simulink model "ESQUEMA"  (R2022b)
settings: Solver=VariableStepAuto  StartTime=0.0  StopTime=inf  RelTol=1e-3
libraries: dsparch4 x12, dspvision x2, dspmathops x1
settings Model: Creator=Core I5  LastModifiedBy=mluser
settings SolverCC: AlgebraicLoopSolver=TrustRegion
settings DataIOCC: ReturnWorkspaceOutputs=off
settings DebuggingCC: UnconnectedInputMsg=warning  UnconnectedOutputMsg=warning  UnconnectedLineMsg=warning  SFMachineParentedDataDiag=warning  ArithmeticOperatorsInVariantConditions=warning
settings ModelReferenceCC: EnableRefExpFcnMdlSchedulingChecks=on
settings SFSimCC: SimUseLocalCustomCode=off  CustomCodeUndefinedFunction=UseInterfaceOnly
settings RTWCC: RTWUseLocalCustomCode=off

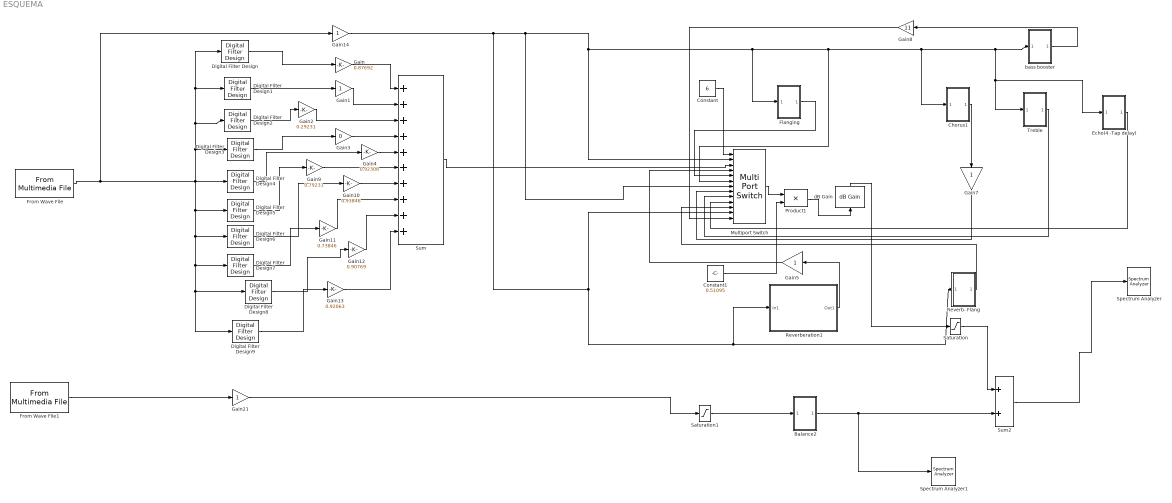
== system ESQUEMA ==
  Balance2 : Subsystem
  "Chorus1 " : Subsystem
  Constant : Constant  Value=6
  Constant1 : Constant  Value=0.51095
  Digital Filter Design{,1..9} (10 alike) : dsparch4/Digital Filter Design  mwdsp_browser_bugfix_var=off
  Echo(4 -Tap delay) : Subsystem
  Flanging : Subsystem
  From Wave File : dspvision/From Multimedia File  inputFilename=/MATLAB Drive/202209180308.wav  readRange=[1 Inf]  loop=on  numPlays=1  outputStreams=Audio only  videoDataType=single  audioDataType=double  inheritSampleTime=on  userDefinedSampleTime=1/30  noAudioOutput=off  isIntensityVideo=off  fourcc=RGB  colorVideoFormat=Separate color signals  outputEOF=off  dataOrg=Column-major  audioFrameSize=256  computeAudioFrameSize=off  outSamplingMode=Frame based
  From Wave File1 : dspvision/From Multimedia File  inputFilename=/MATLAB Drive/09180438.wav  readRange=[1 Inf]  loop=on  numPlays=1  outputStreams=Audio only  videoDataType=single  audioDataType=double  inheritSampleTime=on  userDefinedSampleTime=1/30  noAudioOutput=off  isIntensityVideo=off  fourcc=RGB  colorVideoFormat=Separate color signals  outputEOF=off  dataOrg=Column-major  audioFrameSize=256  computeAudioFrameSize=off  outSamplingMode=Frame based
  Gain : Gain  Gain=0.87692  SaturateOnIntegerOverflow=on  OutDataTypeStr=Inherit: Same as input  ParamDataTypeStr=Inherit: Same as input
  Gain{1,5,7,14,21} (5 alike) : Gain  SaturateOnIntegerOverflow=on  OutDataTypeStr=Inherit: Same as input  ParamDataTypeStr=Inherit: Same as input
  Gain10 : Gain  Gain=0.93846  SaturateOnIntegerOverflow=on  OutDataTypeStr=Inherit: Same as input  ParamDataTypeStr=Inherit: Same as input
  Gain11 : Gain  Gain=0.73846  SaturateOnIntegerOverflow=on  OutDataTypeStr=Inherit: Same as input  ParamDataTypeStr=Inherit: Same as input
  Gain12 : Gain  Gain=0.90769  SaturateOnIntegerOverflow=on  OutDataTypeStr=Inherit: Same as input  ParamDataTypeStr=Inherit: Same as input
  Gain13 : Gain  Gain=0.92063  SaturateOnIntegerOverflow=on  OutDataTypeStr=Inherit: Same as input  ParamDataTypeStr=Inherit: Same as input
  Gain2 : Gain  Gain=0.29231  SaturateOnIntegerOverflow=on  OutDataTypeStr=Inherit: Same as input  ParamDataTypeStr=Inherit: Same as input
  Gain3 : Gain  Gain=0  SaturateOnIntegerOverflow=on  OutDataTypeStr=Inherit: Same as input  ParamDataTypeStr=Inherit: Same as input
  Gain4 : Gain  Gain=0.92308  SaturateOnIntegerOverflow=on  OutDataTypeStr=Inherit: Same as input  ParamDataTypeStr=Inherit: Same as input
  Gain8 : Gain  Gain=11  SaturateOnIntegerOverflow=on  OutDataTypeStr=Inherit: Same as input  ParamDataTypeStr=Inherit: Same as input
  Gain9 : Gain  Gain=0.79231  SaturateOnIntegerOverflow=on  OutDataTypeStr=Inherit: Same as input  ParamDataTypeStr=Inherit: Same as input
  Multiport Switch : MultiPortSwitch  Inputs=12  InputSameDT=off
  Product1 : Product  SaturateOnIntegerOverflow=on  OutDataTypeStr=Inherit: Same as first input
  Reverb- Flang : Subsystem
  Reverberation1 : Subsystem
  Saturation : Saturate  UpperLimit=5  LowerLimit=-5  LinearizeAsGain=off  ZeroCross=off
  Saturation1 : Saturate  UpperLimit=5  LowerLimit=-5  LinearizeAsGain=off  ZeroCross=off
  Spectrum Analyzer : SpectrumAnalyzer
  Spectrum Analyzer1 : SpectrumAnalyzer
  Sum : Sum  Inputs=++++++++++  SaturateOnIntegerOverflow=on
  Sum2 : Sum  SaturateOnIntegerOverflow=on
  Treble : Subsystem
  bass booster : Subsystem
  dB Gain : dspmathops/dB Gain  dB=0.43796  intype=Amplitude
  wires:
  Gain2/1 -> Sum/3
  Gain14/1 -> Multiport Switch/12, Reverberation1/1(In1), Reverb- Flang/1(In1), Multiport Switch/7, Flanging/1(In1), Multiport Switch/6, "Chorus1 "/1(In1), bass booster/1(In1), Treble/1(In1), Echo(4 -Tap delay)/1(In1), Multiport Switch/2
  From Wave File/1 -> Digital Filter Design4/1, Digital Filter Design/1, Digital Filter Design1/1, Digital Filter Design2/1, Digital Filter Design3/1, Digital Filter Design5/1, Digital Filter Design6/1, Digital Filter Design7/1, Digital Filter Design9/1, Digital Filter Design8/1, Gain14/1
  Product1/1 -> dB Gain/1
  Sum/1 -> Multiport Switch/3
  Constant/1 -> Multiport Switch/1
  Constant1/1 -> Product1/2
  Digital Filter Design5/1 -> Gain9/1
  Digital Filter Design1/1 -> Gain1/1
  Digital Filter Design9/1 -> Gain13/1
  dB Gain/1 -> Saturation/1
  Gain/1 -> Sum/1
  Gain9/1 -> Sum/6
  Gain11/1 -> Sum/8
  Digital Filter Design4/1 -> Gain4/1
  Gain1/1 -> Sum/2
  Gain8/1 -> Multiport Switch/13
  Gain13/1 -> Sum/10
  Gain5/1 -> Multiport Switch/4
  Gain3/1 -> Sum/4
  Digital Filter Design7/1 -> Gain11/1
  Gain7/1 -> Multiport Switch/8
  Echo(4 -Tap delay)/1(Out1) -> Multiport Switch/10
  Digital Filter Design8/1 -> Gain12/1
  Reverberation1/1(Out1) -> Gain5/1
  Saturation/1 -> Sum2/1
  Gain12/1 -> Sum/9
  Reverb- Flang/1(Out1) -> Multiport Switch/11
  Digital Filter Design3/1 -> Gain3/1
  bass booster/1(Out1) -> Gain8/1
  Digital Filter Design6/1 -> Gain10/1
  Gain4/1 -> Sum/5
  "Chorus1 "/1(Out1) -> Gain7/1
  Digital Filter Design2/1 -> Gain2/1
  Multiport Switch/1 -> Product1/1
  Treble/1(Out1) -> Multiport Switch/9
  Gain10/1 -> Sum/7
  Flanging/1(Out1) -> Multiport Switch/5
  Digital Filter Design/1 -> Gain/1
  Saturation1/1 -> Balance2/1(In1)
  Gain21/1 -> Saturation1/1
  From Wave File1/1 -> Gain21/1
  Balance2/1(Out1) -> Spectrum Analyzer1/1, Sum2/2
  Sum2/1 -> Spectrum Analyzer/1

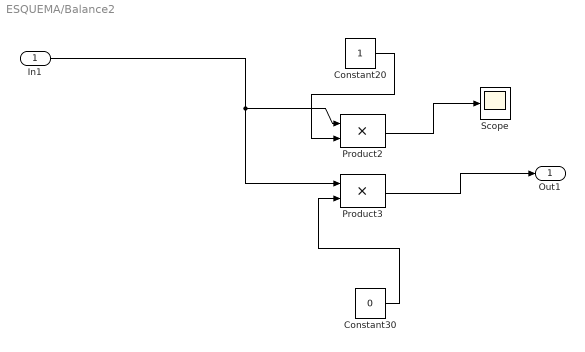
== system ESQUEMA/Balance2 ==
  In1 : Inport
  Constant20 : Constant
  Constant30 : Constant  Value=0
  Product2 : Product  SaturateOnIntegerOverflow=on  OutDataTypeStr=Inherit: Same as first input
  Product3 : Product  SaturateOnIntegerOverflow=on  OutDataTypeStr=Inherit: Same as first input
  Scope : Scope
  Out1 : Outport  VectorParamsAs1DForOutWhenUnconnected=off
  wires:
  Constant20/1 -> Product2/2
  Constant30/1 -> Product3/2
  In1/1 -> Product3/1, Product2/1
  Product3/1 -> Out1/1
  Product2/1 -> Scope/1

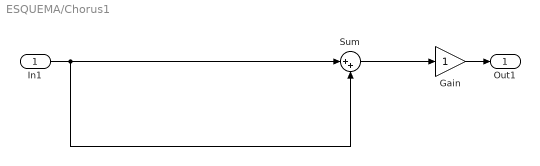
== system ESQUEMA/Chorus1  ==
  In1 : Inport
  Gain : Gain  SaturateOnIntegerOverflow=on  OutDataTypeStr=Inherit: Same as input  ParamDataTypeStr=Inherit: Same as input
  Sum : Sum  Inputs=|++  SaturateOnIntegerOverflow=on
  Out1 : Outport  VectorParamsAs1DForOutWhenUnconnected=off
  wires:
  In1/1 -> Sum/1, Sum/2
  Sum/1 -> Gain/1
  Gain/1 -> Out1/1

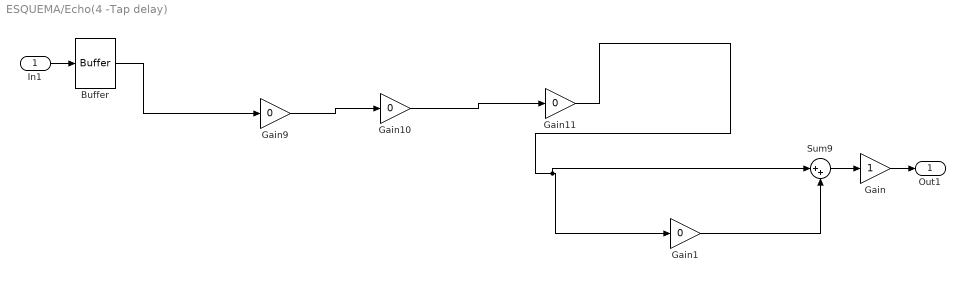
== system ESQUEMA/Echo(4 -Tap delay) ==
  In1 : Inport
  Buffer : Buffer  N=256  ic=100
  Gain : Gain  SaturateOnIntegerOverflow=on  OutDataTypeStr=Inherit: Same as input  ParamDataTypeStr=Inherit: Same as input
  Gain{1,9..11} (4 alike) : Gain  Gain=0  SaturateOnIntegerOverflow=on  OutDataTypeStr=Inherit: Same as input  ParamDataTypeStr=Inherit: Same as input
  Sum9 : Sum  Inputs=|++  SaturateOnIntegerOverflow=on
  Out1 : Outport  VectorParamsAs1DForOutWhenUnconnected=off
  wires:
  Gain10/1 -> Gain11/1
  Gain9/1 -> Gain10/1
  Gain11/1 -> Sum9/1, Gain1/1
  Buffer/1 -> Gain9/1
  Gain1/1 -> Sum9/2
  Sum9/1 -> Gain/1
  In1/1 -> Buffer/1
  Gain/1 -> Out1/1

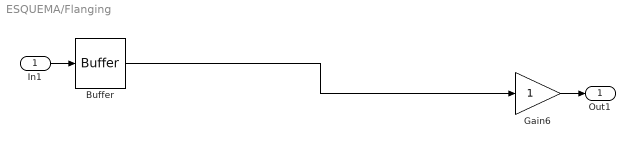
== system ESQUEMA/Flanging ==
  In1 : Inport
  Buffer : Buffer  N=256  ic=100
  Gain6 : Gain  SaturateOnIntegerOverflow=on  OutDataTypeStr=Inherit: Same as input  ParamDataTypeStr=Inherit: Same as input
  Out1 : Outport  VectorParamsAs1DForOutWhenUnconnected=off
  wires:
  Buffer/1 -> Gain6/1
  In1/1 -> Buffer/1
  Gain6/1 -> Out1/1

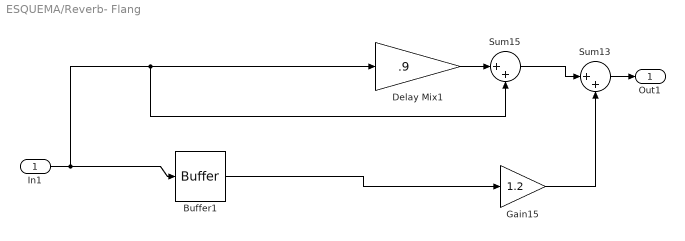
== system ESQUEMA/Reverb- Flang ==
  In1 : Inport
  Buffer1 : Buffer  N=256
  Delay Mix1 : Gain  Gain=.9  SaturateOnIntegerOverflow=on  OutDataTypeStr=Inherit: Same as input  ParamDataTypeStr=Inherit: Same as input
  Gain15 : Gain  Gain=1.2  SaturateOnIntegerOverflow=on  OutDataTypeStr=Inherit: Same as input  ParamDataTypeStr=Inherit: Same as input
  Sum13 : Sum  Inputs=|++  InputSameDT=on  SaturateOnIntegerOverflow=on  OutDataTypeStr=Inherit: Same as first input
  Sum15 : Sum  Inputs=|++  InputSameDT=on  SaturateOnIntegerOverflow=on  OutDataTypeStr=Inherit: Same as first input
  Out1 : Outport  VectorParamsAs1DForOutWhenUnconnected=off
  wires:
  Buffer1/1 -> Gain15/1
  Gain15/1 -> Sum13/2
  Sum15/1 -> Sum13/1
  Delay Mix1/1 -> Sum15/1
  In1/1 -> Delay Mix1/1, Sum15/2, Buffer1/1
  Sum13/1 -> Out1/1

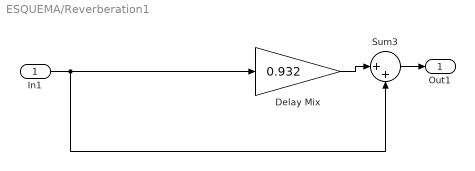
== system ESQUEMA/Reverberation1 ==
  In1 : Inport
  Delay Mix : Gain  Gain=0.932  SaturateOnIntegerOverflow=on  OutDataTypeStr=Inherit: Same as input  ParamDataTypeStr=Inherit: Same as input
  Sum3 : Sum  Inputs=|++  InputSameDT=on  SaturateOnIntegerOverflow=on  OutDataTypeStr=Inherit: Same as first input
  Out1 : Outport  VectorParamsAs1DForOutWhenUnconnected=off
  wires:
  Sum3/1 -> Out1/1
  Delay Mix/1 -> Sum3/1
  In1/1 -> Delay Mix/1, Sum3/2

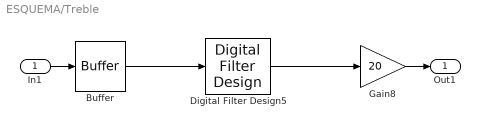
== system ESQUEMA/Treble ==
  In1 : Inport
  Buffer : Buffer  N=256  ic=100
  Digital Filter Design5 : dsparch4/Digital Filter Design  mwdsp_browser_bugfix_var=off
  Gain8 : Gain  Gain=20  SaturateOnIntegerOverflow=on  OutDataTypeStr=Inherit: Same as input  ParamDataTypeStr=Inherit: Same as input
  Out1 : Outport  VectorParamsAs1DForOutWhenUnconnected=off
  wires:
  Buffer/1 -> Digital Filter Design5/1
  Digital Filter Design5/1 -> Gain8/1
  In1/1 -> Buffer/1
  Gain8/1 -> Out1/1

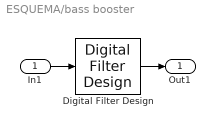
== system ESQUEMA/bass booster ==
  In1 : Inport
  Digital Filter Design : dsparch4/Digital Filter Design  mwdsp_browser_bugfix_var=off
  Out1 : Outport  VectorParamsAs1DForOutWhenUnconnected=off
  wires:
  In1/1 -> Digital Filter Design/1
  Digital Filter Design/1 -> Out1/1
